simulink model "SMC_network"  (R2021a)
settings: Solver=VariableStepAuto  StartTime=0.0  StopTime=5  RelTol=1e-3
values from neighbouring files (symbols this model uses):
  C = 1e-12    [SMCCodes.m]
  eta_d = 1e27    (= 1e+27)    [SMCCodes.m]
  eta_ds = 1e5    (= 100000)    [SMCCodes.m]
  eta_q = 1e27    (= 1e+27)    [SMCCodes.m]
  eta_qs = 1e5    (= 100000)    [SMCCodes.m]
  g = -10e14    (= -1e+15)    [SMCCodes.m]
  gs = -1/Lt    (= -99.6909580301)    [SMCCodes.m]
  L = 100e-3    (= 0.1)    [SMCCodes.m]
  lambda = 1e10    (= 10000000000)    [SMCCodes.m]
  Lf = 10e-3    (= 0.01)    [SMCCodes.m]
  Lg = 0    [SMCCodes.m]
  Ll = 31e-6    (= 3.1e-05)    [SMCCodes.m]
  phi = 0.01    [SMCCodes.m]
  R = 4.33    [SMCCodes.m]
  Rf = 40e-3    (= 0.04)    [SMCCodes.m]
  RL = 0.1    [SMCCodes.m]
  Ts = 0.50e-5    (= 5e-06)    [SMCCodes.m]
undefined symbols (not defined in the file or in its folder): Ion, Lithium, sigbuilder_block
libraries: spsMeanLib x47, spsSeriesRLCBranchLib x23, simulink x22, spsFirstOrderFilterLib x10, spsIGBTDiodeLib x8, pid_lib x8, spsPWMGeneratorDCDCLib x8, spsabctodq0Lib x7, spsThreePhaseVIMeasurementLib x6, spsCurrentMeasurementLib x4, spsDiodeLib x4, spsIGBTLib x4
(part 1 of 3)
settings Model: SimulationMode=accelerator  Creator=Mori  LastModifiedBy=Mori
settings SolverCC: ZeroCrossAlgorithm=Adaptive
settings OptimizationCC: AccelVerboseBuild=on
settings DebuggingCC: MaskedZcDiagnostic=none  IgnoredZcDiagnostic=none  ModelReferenceExtraNoncontSigs=none

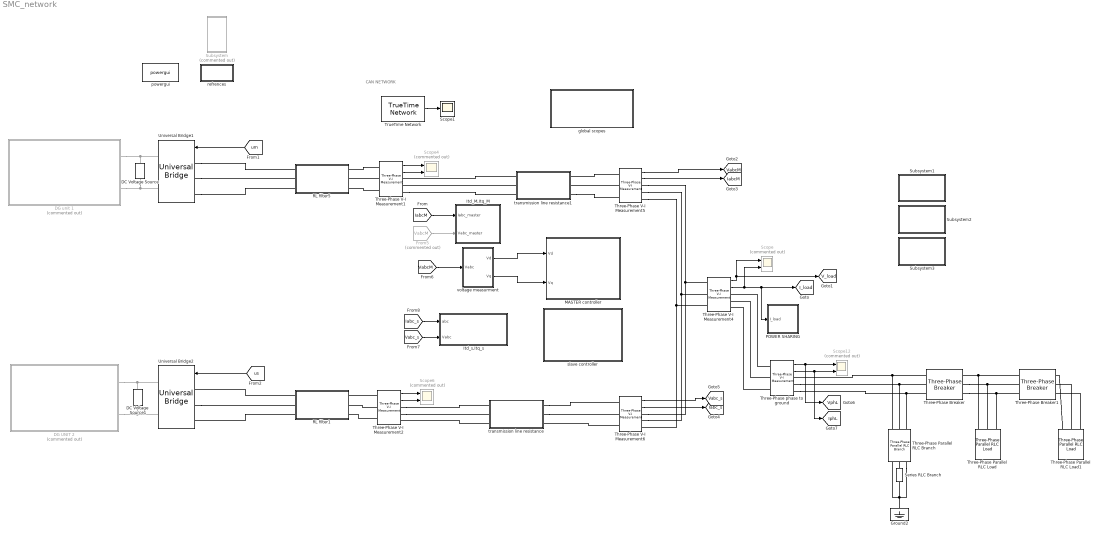
== system SMC_network ==
  note: CAN NETWORK
  DC Voltage Source : spsDCVoltageSourceLib/DC Voltage Source  Amplitude=1000  Measurements=None
  DC Voltage Source1 : spsDCVoltageSourceLib/DC Voltage Source  Amplitude=1000  Measurements=None
  DG UNIT 2 : Subsystem  Commented=on
  DG unit 1 : Subsystem  Commented=on
  From5 : From  Commented=on  GotoTag=VabcM  TagVisibility=global
  Ground2 : spsGroundLib/Ground  LConnTagsString=a
  Itd_M,Itq_M : Subsystem
  Itd_s,Itq_s : Subsystem
  MASTER controller : Subsystem
  POWER SHARING : Subsystem
  RL filter1 : Subsystem
  RL filter5 : Subsystem
  Scope{,4,6,12} (4 alike) : Scope  Commented=on  NumInputPorts=2
  Scope1 : Scope
  Series RLC Branch : spsSeriesRLCBranchLib/Series RLC Branch  LConnTagsString=__new0  RConnTagsString=__new0  BranchType=R  Resistance=0.1  Inductance=1e-3  SetiL0=off  InitialCurrent=0  Capacitance=1e-6  Setx0=off  InitialVoltage=0  Measurements=None
  Subsystem : Subsystem  Commented=on
  Subsystem1 : Subsystem
  Subsystem2 : Subsystem
  Subsystem3 : Subsystem
  Three-Phase Parallel RLC Branch : spsThreePhaseParallelRLCBranchLib/Three-Phase Parallel RLC Branch  LConnTagsString=A|B|C  RConnTagsString=A|B|C  BranchType=RLC  Resistance=R  Inductance=L  Capacitance=C  Measurements=Branch voltages and currents
      settings: SourceProductBaseCode=PS
  Three-Phase Parallel RLC Load : spsThreePhaseParallelRLCLoadLib/Three-Phase Parallel RLC Load  LConnTagsString=A|B|C  Configuration=Y (grounded)  NominalVoltage=380  Vabc=[1e3 1e3 1e3]  Vabcp=[1e3 1e3 1e3]  NominalFrequency=50  UnbalancedPower=off  ActivePower=30e3  InductivePower=5e3  CapacitivePower=0  Pabc=[10e3 9e3 11e3]  QLabc=[100 90 110]  QCabc=[100 90 110]  Pabcp=[10e3 9e3 11e3]  QLabcp=[100 90 110]  QCabcp=[100 90 110]  Measurements=None  LoadType=constant PQ
  Three-Phase Parallel RLC Load1 : spsThreePhaseParallelRLCLoadLib/Three-Phase Parallel RLC Load  LConnTagsString=A|B|C  Configuration=Y (grounded)  NominalVoltage=380  Vabc=[1e3 1e3 1e3]  Vabcp=[1e3 1e3 1e3]  NominalFrequency=50  UnbalancedPower=off  ActivePower=10e3  InductivePower=0  CapacitivePower=0  Pabc=[10e3 9e3 11e3]  QLabc=[100 90 110]  QCabc=[100 90 110]  Pabcp=[10e3 9e3 11e3]  QLabcp=[100 90 110]  QCabcp=[100 90 110]  Measurements=None  LoadType=constant PQ
  Three-Phase V-I Measurement1 : spsThreePhaseVIMeasurementLib/Three-Phase V-I Measurement  VoltageMeasurement=phase-to-phase  SetLabelV=off  LabelV=Vabc  Vpu=off  VpuLL=off  CurrentMeasurement=yes  SetLabelI=off  LabelI=Iabc  Ipu=off  Pbase=100e6  Vbase=500e3  OutputType=Complex  PhasorSimulation=off  PSBequivalent=0
  Three-Phase V-I Measurement2 : spsThreePhaseVIMeasurementLib/Three-Phase V-I Measurement  VoltageMeasurement=phase-to-phase  SetLabelV=off  LabelV=Vabc  Vpu=off  VpuLL=off  CurrentMeasurement=yes  SetLabelI=off  LabelI=Iabc  Ipu=off  Pbase=100e6  Vbase=500e3  OutputType=Complex  PhasorSimulation=off  PSBequivalent=0
  Three-Phase V-I Measurement4 : spsThreePhaseVIMeasurementLib/Three-Phase V-I Measurement  VoltageMeasurement=phase-to-phase  SetLabelV=off  LabelV=Vabc  Vpu=off  VpuLL=off  CurrentMeasurement=yes  SetLabelI=off  LabelI=Iabc  Ipu=off  Pbase=100e6  Vbase=380  OutputType=Complex  PhasorSimulation=off  PSBequivalent=0
  Three-Phase V-I Measurement5 : spsThreePhaseVIMeasurementLib/Three-Phase V-I Measurement  VoltageMeasurement=phase-to-ground  SetLabelV=off  LabelV=Vabc  Vpu=off  VpuLL=off  CurrentMeasurement=yes  SetLabelI=off  LabelI=Iabc  Ipu=off  Pbase=100e6  Vbase=500e3  OutputType=Complex  PhasorSimulation=off  PSBequivalent=0
  Three-Phase V-I Measurement6 : spsThreePhaseVIMeasurementLib/Three-Phase V-I Measurement  VoltageMeasurement=phase-to-ground  SetLabelV=off  LabelV=Vabc  Vpu=off  VpuLL=off  CurrentMeasurement=yes  SetLabelI=off  LabelI=Iabc  Ipu=off  Pbase=100e6  Vbase=500e3  OutputType=Complex  PhasorSimulation=off  PSBequivalent=0
  Three-Phase phase to ground : spsThreePhaseVIMeasurementLib/Three-Phase V-I Measurement  VoltageMeasurement=phase-to-ground  SetLabelV=off  LabelV=Vabc  Vpu=off  VpuLL=off  CurrentMeasurement=yes  SetLabelI=off  LabelI=Iabc  Ipu=off  Pbase=100e6  Vbase=500e3  OutputType=Complex  PhasorSimulation=off  PSBequivalent=0
  Three-Phase Breaker : spsThreePhaseBreakerLib/Three-Phase Breaker  InitialState=open  SwitchA=on  SwitchB=on  SwitchC=on  SwitchTimes=[1,4]  External=off  BreakerResistance=0.001  SnubberResistance=1e6  SnubberCapacitance=inf  Measurements=None
  Three-Phase Breaker1 : spsThreePhaseBreakerLib/Three-Phase Breaker  InitialState=open  SwitchA=on  SwitchB=on  SwitchC=on  SwitchTimes=[2,3]  External=off  BreakerResistance=0.001  SnubberResistance=1e6  SnubberCapacitance=inf  Measurements=None
  TrueTime Network : truetime/TrueTime Network  nwtype=CSMA/AMP (CAN)  nwnbr=1  nnodes=2  rate=10000000  minsize=512  lossprob=0  seed=0  bandwidths=[0.5 0.5]  slotsize=512  schedule=[1 1 2]  memsize=80000  buftype=Common buffer  overflow=Retransmit  dynSchedule=0  miniSlotSize=0  NIT=0  QSortMode=FIFO  sync=0  irtSchedule=0  nrtLength=0  nodeGraph=0  scheduleoutput=on
  Universal Bridge1 : spsUniversalBridgeLib/Universal Bridge  Arms=3  SnubberResistance=1e3  SnubberCapacitance=inf  Device=MOSFET / Diodes  Ron=1e-3  Lon=0  ForwardVoltages="[  0  0  ]"  ForwardVoltage=0  GTOparameters=[ 10e-6 , 20e-6 ]  IGBTparameters=[ 1e-6 , 2e-6 ]  Measurements=None  Measurements_2=None  converterType=Rectifier
  Universal Bridge2 : spsUniversalBridgeLib/Universal Bridge  Arms=3  SnubberResistance=1e3  SnubberCapacitance=inf  Device=MOSFET / Diodes  Ron=1e-3  Lon=0  ForwardVoltages="[  0  0  ]"  ForwardVoltage=0  GTOparameters=[ 10e-6 , 20e-6 ]  IGBTparameters=[ 1e-6 , 2e-6 ]  Measurements=None  Measurements_2=None  converterType=Rectifier
  global scopes : Subsystem
  powergui : spspowerguiLib/powergui  Priority=1  SimulationMode=Discrete  SampleTime=Ts  frequency=60  Iterations=50  frequencyindice=0  Pbase=100e6  ErrMax=1e-4  UnitsV=kV  UnitsW=MW  buscounter=0  FunctionMessages=off  echomessages=off  EnableUseOfTLC=off  CurrentSourceSwitches=off  DisableSnubberDevices=off  DisableRonSwitches=off  DisableVfSwitches=off  DisplayEquations=off  AutomaticDiscreteSolvers=off  SolverType=Tustin/Backward Euler (TBE)  Interpol=off  ExternalGateDelay=off  methode=off  Ts=100  x0status=blocks  SPID=on  SwTol=0  HookPort=off  NonlinearTolerance=1e-4  nMaxIteration=100  ContinueOnMaxIteration=off  RestoreLinks=warning  ResistiveCurrentMeasurement=off  Frange=[0:2:500]  Ylog=off  Xlog=on  ShowGrid=off  save=off  variable=ZData  structure=0  ZoomFFT=off  StartTime=0.0  cycles=1  DisplayStyle=1  fundamental=60  FreqAxis=off  MaxFrequency=1000  frequencyindicesteady=1  RmsSteady=1  display=off
  refrences : Subsystem
  "slave controller " : Subsystem
  transmission line resistance : Subsystem
  transmission line resistance1 : Subsystem
  voltage measurment : Subsystem
  tag scope: I_load=global, IabcM=global, Iabc_s=global, IphL=global, V_load=global, VabcM=global, Vabc_s=global, VphL=global
  wires:
  Three-Phase V-I Measurement4/2 -> Scope/2, POWER SHARING/1(I_load), [I_load]
  Three-Phase V-I Measurement4/1 -> Scope/1, [V_load]
  Three-Phase phase to ground/1 -> [VphL], Scope12/1
  Three-Phase phase to ground/2 -> [IphL], Scope12/2
  [VabcM] -> voltage measurment/1(Vabc)
  [us] -> Universal Bridge2/1
  [um] -> Universal Bridge1/1
  From5/1 -> Itd_M,Itq_M/2(Vabc_master)
  [IabcM] -> Itd_M,Itq_M/1(Iabc_master)
  [Iabc_s] -> Itd_s,Itq_s/1(abc)
  voltage measurment/2(Vq) -> MASTER controller/2(Vq)
  voltage measurment/1(Vd) -> MASTER controller/1(Vd)
  [Vabc_s] -> Itd_s,Itq_s/2(Vabc)
  Three-Phase V-I Measurement1/2 -> Scope4/2
  Three-Phase V-I Measurement1/1 -> Scope4/1
  Three-Phase V-I Measurement2/1 -> Scope6/1
  Three-Phase V-I Measurement2/2 -> Scope6/2
  Three-Phase V-I Measurement6/1 -> [Vabc_s]
  Three-Phase V-I Measurement6/2 -> [Iabc_s]
  Three-Phase V-I Measurement5/1 -> [VabcM]
  Three-Phase V-I Measurement5/2 -> [IabcM]
  TrueTime Network/1 -> Scope1/1
  connections:
  Three-Phase Parallel RLC Branch/RConn3 -- Ground2/LConn1 -- Three-Phase Parallel RLC Branch/RConn1 -- Series RLC Branch/RConn1
  Three-Phase V-I Measurement1/LConn1 -- RL filter5/RConn1
  Three-Phase V-I Measurement1/LConn3 -- RL filter5/RConn3
  Universal Bridge1/LConn1 -- RL filter5/LConn1
  Universal Bridge1/LConn3 -- RL filter5/LConn3
  transmission line resistance1/LConn2 -- Three-Phase V-I Measurement1/RConn2
  Universal Bridge1/LConn2 -- RL filter5/LConn2
  Three-Phase V-I Measurement2/RConn1 -- transmission line resistance/LConn1
  Three-Phase V-I Measurement1/LConn2 -- RL filter5/RConn2
  transmission line resistance/LConn3 -- Three-Phase V-I Measurement2/RConn3
  RL filter1/LConn3 -- Universal Bridge2/LConn3
  Three-Phase V-I Measurement2/LConn2 -- RL filter1/RConn2
  RL filter1/LConn1 -- Universal Bridge2/LConn1
  Universal Bridge2/LConn2 -- RL filter1/LConn2
  Three-Phase V-I Measurement2/LConn3 -- RL filter1/RConn3
  Three-Phase V-I Measurement2/LConn1 -- RL filter1/RConn1
  Three-Phase phase to ground/RConn3 -- Three-Phase Parallel RLC Branch/LConn3 -- Three-Phase Breaker/LConn3
  Three-Phase phase to ground/RConn2 -- Three-Phase Parallel RLC Branch/LConn2 -- Three-Phase Breaker/LConn2
  Three-Phase Breaker/LConn1 -- Three-Phase Parallel RLC Branch/LConn1 -- Three-Phase phase to ground/RConn1
  Series RLC Branch/LConn1 -- Three-Phase Parallel RLC Branch/RConn2
  Three-Phase V-I Measurement1/RConn3 -- transmission line resistance1/LConn3
  Three-Phase V-I Measurement2/RConn2 -- transmission line resistance/LConn2
  transmission line resistance1/LConn1 -- Three-Phase V-I Measurement1/RConn1
  Three-Phase V-I Measurement4/LConn2 -- Three-Phase V-I Measurement6/RConn2 -- Three-Phase V-I Measurement5/RConn2
  transmission line resistance1/RConn3 -- Three-Phase V-I Measurement5/LConn3
  Three-Phase V-I Measurement4/LConn1 -- Three-Phase V-I Measurement6/RConn1 -- Three-Phase V-I Measurement5/RConn1
  Three-Phase V-I Measurement5/RConn3 -- Three-Phase V-I Measurement4/LConn3 -- Three-Phase V-I Measurement6/RConn3
  Three-Phase V-I Measurement5/LConn2 -- transmission line resistance1/RConn2
  Three-Phase V-I Measurement5/LConn1 -- transmission line resistance1/RConn1
  Three-Phase V-I Measurement6/LConn3 -- transmission line resistance/RConn3
  transmission line resistance/RConn2 -- Three-Phase V-I Measurement6/LConn2
  transmission line resistance/RConn1 -- Three-Phase V-I Measurement6/LConn1
  Three-Phase Parallel RLC Load/LConn1 -- Three-Phase Breaker1/LConn1 -- Three-Phase Breaker/RConn1
  Three-Phase Breaker/RConn2 -- Three-Phase Breaker1/LConn2 -- Three-Phase Parallel RLC Load/LConn2
  Three-Phase Breaker/RConn3 -- Three-Phase Breaker1/LConn3 -- Three-Phase Parallel RLC Load/LConn3
  Three-Phase phase to ground/LConn1 -- Three-Phase V-I Measurement4/RConn1
  Three-Phase phase to ground/LConn2 -- Three-Phase V-I Measurement4/RConn2
  Three-Phase phase to ground/LConn3 -- Three-Phase V-I Measurement4/RConn3
  Three-Phase Parallel RLC Load1/LConn1 -- Three-Phase Breaker1/RConn1
  Three-Phase Parallel RLC Load1/LConn2 -- Three-Phase Breaker1/RConn2
  Three-Phase Parallel RLC Load1/LConn3 -- Three-Phase Breaker1/RConn3
  DG unit 1/RConn1 -- DC Voltage Source/RConn1 -- Universal Bridge1/RConn1
  DG unit 1/RConn2 -- DC Voltage Source/LConn1 -- Universal Bridge1/RConn2
  DG UNIT 2/RConn1 -- DC Voltage Source1/RConn1 -- Universal Bridge2/RConn1
  DG UNIT 2/RConn2 -- DC Voltage Source1/LConn1 -- Universal Bridge2/RConn2

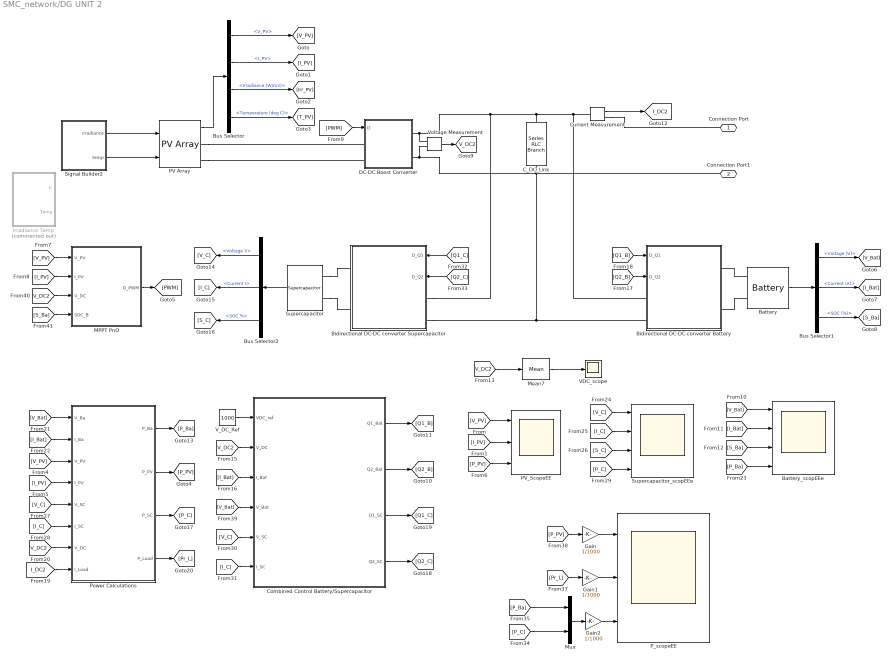
== system SMC_network/DG UNIT 2 ==
  Battery : spsBatteryLib/Battery  BatType=Lithium-Ion  ShowTempParam=off  ThermalPreset=no  ShowAgeParam=off  NomV=750  NomQ=21  SOC=50  Batt_Tr=0.1  PresetModel=on  MaxQ=21  MinV=562.5  FullV=872.9904  Dis_rate=9.1304  R=0.35714  Normal_OP=18.9913  expZone="[810.2894      1.031739]"  current=[9.5 20 28]  Units=Time  Tci=20  NomT=20  T2=-30  MaxQ2=4.8  FullV2=7.1  Normal_OP2=5.655  expZone2="[6.58           1]"  Rca=0.6  ti=2000  Dp=0  Neq0=0  Tsim=1e6  Ta1=25  Qeol=5.4*0.9  Reol=0.013333*1.2  Char_age=[2.3478, 3]  Dis_age=[2.3478, 10]  N1=1500  N2=10500  N3=1000  N4=1400  Ta2=45  N5=950
  "Battery_scopEEe " : Scope  NumInputPorts=4
  Bidirectional DC-DC converter Battery : Subsystem
  Bidirectional DC-DC converter Supercapacitor : Subsystem
  Bus Selector : BusSelector  OutputSignals=V_PV,I_PV,Irradiance (W/m2),Temperature (deg C)
  Bus Selector1 : BusSelector  OutputSignals=Voltage (V),Current (A),SOC (%)
  Bus Selector2 : BusSelector  OutputSignals=Voltage V,Current I,SOC %
  C_DC_Link : spsSeriesRLCBranchLib/Series RLC Branch  LConnTagsString=__new0  RConnTagsString=__new0  BranchType=C  Resistance=1  Inductance=1e-3  SetiL0=off  InitialCurrent=0  Capacitance=500e-6  Setx0=off  InitialVoltage=0  Measurements=None
  Combined Control Battery/Supercapacitor : Subsystem
  Current Measurement : spsCurrentMeasurementLib/Current Measurement  PhasorSimulation=off  OutputType=Complex  PSBequivalent=0
  DC-DC Boost Converter : Subsystem
  Gain : Gain  Gain=1/1000
  Gain1 : Gain  Gain=1/1000
  Gain2 : Gain  Gain=1/1000
  Irradiance Temp : Subsystem  Tag=STV Subsys  Commented=on  LoadFcn=sigbuilder_block('load');  StartFcn=sigbuilder_block('start');  StopFcn=sigbuilder_block('stop');  ClipboardFcn=sigbuilder_block('clipboard');  mask(Sigbuilder block){tuvar=[0:10]}
      mask help: Sigbuilder GUI
      mask init:
      | if ~strcmp(get_param(bdroot(gcbh),'SimulationStatus'),'stopped') tuvar = sigbuilder_block('maskInit'); end
      settings: CopyFcn=sigbuilder_block('copy');  DeleteFcn=sigbuilder_block('delete');  ModelCloseFcn=sigbuilder_block('modelClose');  PreSaveFcn=sigbuilder_block('preSave');  PauseFcn=sigbuilder_block('pause')  ContinueFcn=sigbuilder_block('continue')  NameChangeFcn=sigbuilder_block('namechange');  OpenFcn=sigbuilder_block('open',[216.75 117 531.75 395.25 ]);  CloseFcn=sigbuilder_block('close');
      mask Display: plot(0, 0, 100, 100,[2, 2, 32, 32, 2], [68, 8, 8, 68, 68],[32, 2], [38, 38], [32, 19, 2],[53, 60, 44], [32, 17, 17, 2],[16, 16, 31, 31]);txt = getActiveGroup(gcbh);text(2, 100, txt,'verticalAlignment', 'top');
  MPPT PnO : Subsystem
  Mean7 : spsMeanLib/Mean  Freq=60  Vinit=0  Ts=0
  Mux : Mux  Inputs=2
  PV Array : spsPVArrayLib/PV Array  Npar=3  Nser=30  PlotType=array @ 25 deg.C & specified irradiances  S_vec="[ 1000 800 500  250 ]"  Temp_C_vec="[0 25 50  ]"  ModuleName=Yingli Energy (China) YL250C-30b  PlotWhenSelected=on  Pm=252.815  Ncell=60  Voc=37.6  Isc=9.1  Vm=29.5  Im=8.57  beta_Voc_pc=-0.3  alpha_Isc_pc=0.044  beta_Voc=-0.1128  alpha_Isc=0.004004  IL=9.111  I0=3.084e-11  nI=0.92381  Rsh=475.5958  Rs=0.45532  RobustModel=off  RobustCellTemperature=313.3991  BAL=on  Tc=Tc  Tfilter=5e-5
  PV_ScopeEE : Scope  NumInputPorts=3
  P_scopeEE : Scope  NumInputPorts=3
  Power Calculations : Subsystem
  Signal Builder2 : Subsystem  Tag=STV Subsys  LoadFcn=sigbuilder_block('load');  StartFcn=sigbuilder_block('start');  StopFcn=sigbuilder_block('stop');  ClipboardFcn=sigbuilder_block('clipboard');  mask(Sigbuilder block){tuvar=[0:10]}
      mask help: Simulink:masks:SigbuilderBlock_MD
      mask init:
      | if ~strcmp(get_param(bdroot(gcbh),'SimulationStatus'),'stopped') tuvar = sigbuilder_block('maskInit'); end
      settings: CopyFcn=sigbuilder_block('copy');  DeleteFcn=sigbuilder_block('delete');  ModelCloseFcn=sigbuilder_block('modelClose');  PreSaveFcn=sigbuilder_block('preSave');  PauseFcn=sigbuilder_block('pause');  ContinueFcn=sigbuilder_block('continue');  NameChangeFcn=sigbuilder_block('namechange');  OpenFcn=sigbuilder_block('open',[6 0 1012.5 477.75 ]);  CloseFcn=sigbuilder_block('close');
      mask Display: plot(0, 0, 100, 100,[2, 2, 32, 32, 2], [68, 8, 8, 68, 68],[32, 2], [38, 38], [32, 19, 2],[53, 60, 44], [32, 17, 17, 2],[16, 16, 31, 31]);txt = getActiveGroup(gcbh);text(2, 100, txt,'verticalAlignment', 'top');
  Supercapacitor : spsSupercapacitorLib/Supercapacitor  C=250  Rdc=0.0028  Voltage=820  Ns=1  Np=10  Vinit=820  Temp=25  PresetModel=on  EstParam=off  Nc=1  r=1e-9  epsilon=6.0208e-10  Ich=10  Vstern="[0.161  2.7  7.8]"  Self_dis=on  Ioc=10  Vself="[720  710  701  689]"  demandeplot=off  I=[10 20 100 500]  Units=sec  Vmax=0  If=0  deltaV=0  alpha=0  sec=0
      settings: SourceProductBaseCode=PS
  Supercapacitor_scopEEe : Scope  NumInputPorts=4
  VDC_scope : Scope
  V_DC_Ref : Constant  Value=1000
  Voltage Measurement : spsVoltageMeasurementLib/Voltage Measurement  PhasorSimulation=off  OutputType=Complex  PSBequivalent=0
  Connection Port : PMIOPort  Side=Right
  Connection Port1 : PMIOPort  Port=2  Side=Right
  tag scope: I_DC2=global, V_DC2=global
  wires:
  [P_C] -> Mux/2
  Mux/1 -> Gain2/1
  [P_Ba] -> "Battery_scopEEe "/4
  Mean7/1 -> VDC_scope/1
  [P_Ba] -> Mux/1
  [Pr_L] -> Gain1/1
  [I_Bat] -> Power Calculations/2(I_Ba)
  [P_PV] -> Gain/1
  [I_PV] -> PV_ScopeEE/2
  [V_PV] -> PV_ScopeEE/1
  [I_DC2] -> Power Calculations/8(I_Load)
  [V_Bat] -> Combined Control Battery/Supercapacitor/4(V_Bat)
  Power Calculations/3(P_SC) -> [P_C]
  [V_PV] -> Power Calculations/3(V_PV)
  V_DC_Ref/1 -> Combined Control Battery/Supercapacitor/1(VDC_ref)
  [I_Bat] -> Combined Control Battery/Supercapacitor/3(I_Bat)
  [PWM] -> DC-DC Boost Converter/1(D)
  Bus Selector2/3 -> [S_C]  "<SOC %>"
  [V_DC2] -> Power Calculations/7(V_DC)
  [V_Bat] -> "Battery_scopEEe "/1
  Power Calculations/1(P_Ba) -> [P_Ba]
  [I_C] -> Combined Control Battery/Supercapacitor/6(I_SC)
  [I_Bat] -> "Battery_scopEEe "/2
  Power Calculations/4(P_Load) -> [Pr_L]
  [V_DC2] -> Mean7/1
  [V_PV] -> MPPT PnO/1(V_PV)
  [I_C] -> Power Calculations/6(I_SC)
  [P_PV] -> PV_ScopeEE/3
  [V_Bat] -> Power Calculations/1(V_Ba)
  Current Measurement/1 -> [I_DC2]
  [S_C] -> Supercapacitor_scopEEe/3
  Combined Control Battery/Supercapacitor/3(Q1_SC) -> [Q1_C]
  [S_Ba] -> "Battery_scopEEe "/3
  Bus Selector2/2 -> [I_C]  "<Current I>"
  [P_C] -> Supercapacitor_scopEEe/4
  [V_C] -> Combined Control Battery/Supercapacitor/5("V_SC ")
  Supercapacitor/1 -> Bus Selector2/1
  Bus Selector2/1 -> [V_C]  "<Voltage V>"
  Combined Control Battery/Supercapacitor/2(Q2_Bat) -> [Q2_B]
  [S_Ba] -> MPPT PnO/4(SOC_B)
  [I_C] -> Supercapacitor_scopEEe/2
  [Q2_C] -> Bidirectional DC-DC converter Supercapacitor/2(D_Q2)
  [V_DC2] -> MPPT PnO/3(V_DC)
  [Q1_C] -> Bidirectional DC-DC converter Supercapacitor/1(D_Q1)
  PV Array/1 -> Bus Selector/1
  Bus Selector1/3 -> [S_Ba]  "<SOC (%)>"
  [Q2_B] -> Bidirectional DC-DC converter Battery/2(D_Q2)
  Voltage Measurement/1 -> [V_DC2]
  [Q1_B] -> Bidirectional DC-DC converter Battery/1(D_Q1)
  Battery/1 -> Bus Selector1/1
  [V_DC2] -> Combined Control Battery/Supercapacitor/2(V_DC)
  Bus Selector1/2 -> [I_Bat]  "<Current (A)>"
  Bus Selector1/1 -> [V_Bat]  "<Voltage (V)>"
  [V_C] -> Power Calculations/5(V_SC)
  Bus Selector/4 -> [T_PV]  "<Temperature (deg C)>"
  Combined Control Battery/Supercapacitor/1(Q1_Bat) -> [Q1_B]
  MPPT PnO/1(D_PWM) -> [PWM]
  Bus Selector/3 -> [Irr_PV]  "<Irradiance (W/m2)>"
  Power Calculations/2(P_PV) -> [P_PV]
  [I_PV] -> Power Calculations/4(I_PV)
  Combined Control Battery/Supercapacitor/4(Q2_SC) -> [Q2_C]
  [I_PV] -> MPPT PnO/2(I_PV)
  Bus Selector/2 -> [I_PV]  "<I_PV>"
  Bus Selector/1 -> [V_PV]  "<V_PV>"
  [V_C] -> Supercapacitor_scopEEe/1
  Signal Builder2/1(irradiance) -> PV Array/1
  Signal Builder2/2(temp) -> PV Array/2
  Gain/1 -> P_scopeEE/1
  Gain1/1 -> P_scopeEE/2
  Gain2/1 -> P_scopeEE/3
  connections:
  Bidirectional DC-DC converter Supercapacitor/LConn1 -- Voltage Measurement/LConn1 -- DC-DC Boost Converter/RConn1 -- Bidirectional DC-DC converter Battery/LConn1 -- Current Measurement/LConn1 -- C_DC_Link/LConn1
  Bidirectional DC-DC converter Supercapacitor/LConn2 -- Bidirectional DC-DC converter Battery/LConn2 -- Connection Port1/RConn1 -- C_DC_Link/RConn1 -- Voltage Measurement/LConn2 -- DC-DC Boost Converter/RConn2
  Current Measurement/RConn1 -- Connection Port/RConn1
  Battery/LConn2 -- Bidirectional DC-DC converter Battery/RConn2
  Battery/LConn1 -- Bidirectional DC-DC converter Battery/RConn1
  PV Array/RConn1 -- DC-DC Boost Converter/LConn1
  Supercapacitor/LConn1 -- Bidirectional DC-DC converter Supercapacitor/RConn1
  PV Array/RConn2 -- DC-DC Boost Converter/LConn2
  Supercapacitor/LConn2 -- Bidirectional DC-DC converter Supercapacitor/RConn2

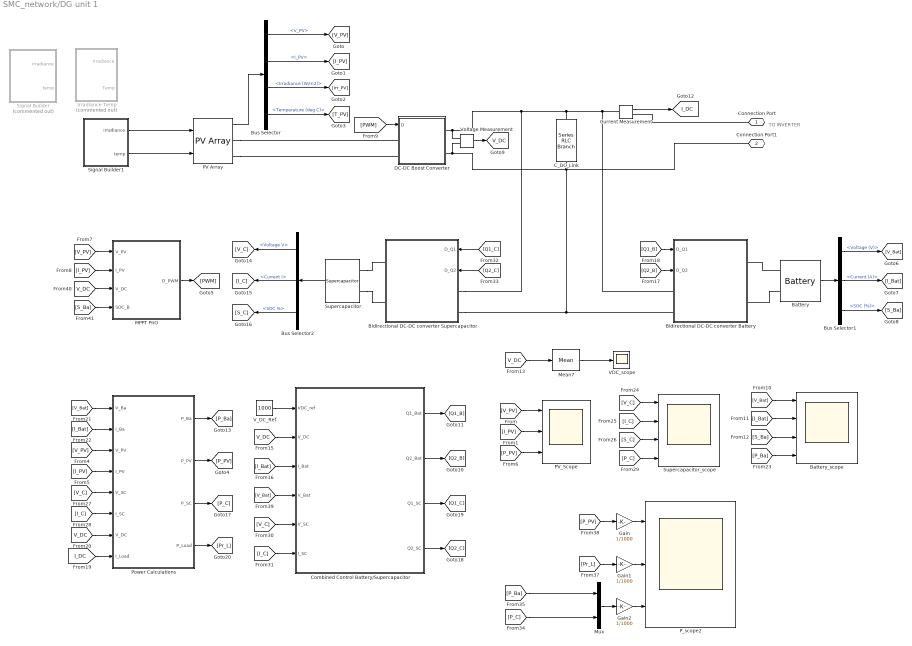
== system SMC_network/DG unit 1 ==
  note: TO INVERTER
  Battery : spsBatteryLib/Battery  BatType=Lithium-Ion  ShowTempParam=off  ThermalPreset=no  ShowAgeParam=off  NomV=750  NomQ=40  SOC=50  Batt_Tr=0.1  PresetModel=on  MaxQ=40  MinV=562.5  FullV=872.9904  Dis_rate=17.3913  R=0.1875  Normal_OP=36.1739  expZone="[810.2894      1.965217]"  current=[17.5 35 52]  Units=Time  Tci=20  NomT=20  T2=-30  MaxQ2=4.8  FullV2=7.1  Normal_OP2=5.655  expZone2="[6.58           1]"  Rca=0.6  ti=2000  Dp=0  Neq0=0  Tsim=1e6  Ta1=25  Qeol=5.4*0.9  Reol=0.013333*1.2  Char_age=[2.3478, 3]  Dis_age=[2.3478, 10]  N1=1500  N2=10500  N3=1000  N4=1400  Ta2=45  N5=950
  "Battery_scope " : Scope  NumInputPorts=4
  Bidirectional DC-DC converter Battery : Subsystem
  Bidirectional DC-DC converter Supercapacitor : Subsystem
  Bus Selector : BusSelector  OutputSignals=V_PV,I_PV,Irradiance (W/m2),Temperature (deg C)
  Bus Selector1 : BusSelector  OutputSignals=Voltage (V),Current (A),SOC (%)
  Bus Selector2 : BusSelector  OutputSignals=Voltage V,Current I,SOC %
  C_DC_Link : spsSeriesRLCBranchLib/Series RLC Branch  LConnTagsString=__new0  RConnTagsString=__new0  BranchType=C  Resistance=1  Inductance=1e-3  SetiL0=off  InitialCurrent=0  Capacitance=500e-6  Setx0=off  InitialVoltage=0  Measurements=None
  Combined Control Battery/Supercapacitor : Subsystem
  Current Measurement : spsCurrentMeasurementLib/Current Measurement  PhasorSimulation=off  OutputType=Complex  PSBequivalent=0
  DC-DC Boost Converter : Subsystem
  Gain : Gain  Gain=1/1000
  Gain1 : Gain  Gain=1/1000
  Gain2 : Gain  Gain=1/1000
  Irradiance Temp : Subsystem  Tag=STV Subsys  Commented=on  LoadFcn=sigbuilder_block('load');  StartFcn=sigbuilder_block('start');  StopFcn=sigbuilder_block('stop');  ClipboardFcn=sigbuilder_block('clipboard');  mask(Sigbuilder block){tuvar=[0:10]}
      mask help: Sigbuilder GUI
      mask init:
      | if ~strcmp(get_param(bdroot(gcbh),'SimulationStatus'),'stopped') tuvar = sigbuilder_block('maskInit'); end
      settings: CopyFcn=sigbuilder_block('copy');  DeleteFcn=sigbuilder_block('delete');  ModelCloseFcn=sigbuilder_block('modelClose');  PreSaveFcn=sigbuilder_block('preSave');  PauseFcn=sigbuilder_block('pause')  ContinueFcn=sigbuilder_block('continue')  NameChangeFcn=sigbuilder_block('namechange');  OpenFcn=sigbuilder_block('open',[0 0 1024.5 518.25 ]);  CloseFcn=sigbuilder_block('close');
      mask Display: plot(0, 0, 100, 100,[2, 2, 32, 32, 2], [68, 8, 8, 68, 68],[32, 2], [38, 38], [32, 19, 2],[53, 60, 44], [32, 17, 17, 2],[16, 16, 31, 31]);txt = getActiveGroup(gcbh);text(2, 100, txt,'verticalAlignment', 'top');
  MPPT PnO : Subsystem
  Mean7 : spsMeanLib/Mean  Freq=60  Vinit=0  Ts=0
  Mux : Mux  Inputs=2
  PV Array : spsPVArrayLib/PV Array  Npar=6  Nser=30  PlotType=array @ 25 deg.C & specified irradiances  S_vec="[ 1000 800 500  250 ]"  Temp_C_vec="[0 25 50  ]"  ModuleName=Yingli Energy (China) YL250P-29b  PlotWhenSelected=on  Pm=250.496  Ncell=60  Voc=38.4  Isc=8.79  Vm=30.4  Im=8.24  beta_Voc_pc=-0.337  alpha_Isc_pc=0.0438  beta_Voc=-0.12941  alpha_Isc=0.00385  IL=8.8005  I0=1.272e-10  nI=0.99849  Rsh=362.5163  Rs=0.42475  RobustModel=off  RobustCellTemperature=313.3991  BAL=on  Tc=Tc  Tfilter=5e-5
  PV_Scope : Scope  NumInputPorts=3
  P_scope2 : Scope  NumInputPorts=3
  Power Calculations : Subsystem
  Signal Builder : Subsystem  Tag=STV Subsys  Commented=on  LoadFcn=sigbuilder_block('load');  StartFcn=sigbuilder_block('start');  StopFcn=sigbuilder_block('stop');  ClipboardFcn=sigbuilder_block('clipboard');  mask(Sigbuilder block){tuvar=[0:10]}
      mask help: Simulink:masks:SigbuilderBlock_MD
      mask init:
      | if ~strcmp(get_param(bdroot(gcbh),'SimulationStatus'),'stopped') tuvar = sigbuilder_block('maskInit'); end
      settings: CopyFcn=sigbuilder_block('copy');  DeleteFcn=sigbuilder_block('delete');  ModelCloseFcn=sigbuilder_block('modelClose');  PreSaveFcn=sigbuilder_block('preSave');  PauseFcn=sigbuilder_block('pause');  ContinueFcn=sigbuilder_block('continue');  NameChangeFcn=sigbuilder_block('namechange');  OpenFcn=sigbuilder_block('open',[6 0 1012.5 477.75 ]);  CloseFcn=sigbuilder_block('close');
      mask Display: plot(0, 0, 100, 100,[2, 2, 32, 32, 2], [68, 8, 8, 68, 68],[32, 2], [38, 38], [32, 19, 2],[53, 60, 44], [32, 17, 17, 2],[16, 16, 31, 31]);txt = getActiveGroup(gcbh);text(2, 100, txt,'verticalAlignment', 'top');
  Signal Builder1 : Subsystem  Tag=STV Subsys  LoadFcn=sigbuilder_block('load');  StartFcn=sigbuilder_block('start');  StopFcn=sigbuilder_block('stop');  ClipboardFcn=sigbuilder_block('clipboard');  mask(Sigbuilder block){tuvar=[0:10]}
      mask help: Simulink:masks:SigbuilderBlock_MD
      mask init:
      | if ~strcmp(get_param(bdroot(gcbh),'SimulationStatus'),'stopped') tuvar = sigbuilder_block('maskInit'); end
      settings: CopyFcn=sigbuilder_block('copy');  DeleteFcn=sigbuilder_block('delete');  ModelCloseFcn=sigbuilder_block('modelClose');  PreSaveFcn=sigbuilder_block('preSave');  PauseFcn=sigbuilder_block('pause');  ContinueFcn=sigbuilder_block('continue');  NameChangeFcn=sigbuilder_block('namechange');  OpenFcn=sigbuilder_block('open',[6 0 1012.5 477.75 ]);  CloseFcn=sigbuilder_block('close');
      mask Display: plot(0, 0, 100, 100,[2, 2, 32, 32, 2], [68, 8, 8, 68, 68],[32, 2], [38, 38], [32, 19, 2],[53, 60, 44], [32, 17, 17, 2],[16, 16, 31, 31]);txt = getActiveGroup(gcbh);text(2, 100, txt,'verticalAlignment', 'top');
  Supercapacitor : spsSupercapacitorLib/Supercapacitor  C=350  Rdc=0.003  Voltage=820  Ns=1  Np=12  Vinit=820  Temp=25  PresetModel=on  EstParam=off  Nc=1  r=1e-9  epsilon=6.0208e-10  Ich=10  Vstern="[0.161  2.7  7.8]"  Self_dis=on  Ioc=10  Vself="[720  710  701  689]"  demandeplot=off  I="[40 50 100  500]"  Units=sec  Vmax=0  If=0  deltaV=0  alpha=0  sec=0
      settings: SourceProductBaseCode=PS
  Supercapacitor_scope : Scope  NumInputPorts=4
  VDC_scope : Scope
  V_DC_Ref : Constant  Value=1000
  Voltage Measurement : spsVoltageMeasurementLib/Voltage Measurement  PhasorSimulation=off  OutputType=Complex  PSBequivalent=0
  Connection Port : PMIOPort  Side=Right
  Connection Port1 : PMIOPort  Port=2  Side=Right
  tag scope: I_DC=global, V_DC=global
  wires:
  [P_C] -> Mux/2
  Bus Selector/2 -> [I_PV]  "<I_PV>"
  [P_PV] -> PV_Scope/3
  Current Measurement/1 -> [I_DC]
  Bus Selector2/1 -> [V_C]  "<Voltage V>"
  [PWM] -> DC-DC Boost Converter/1(D)
  Bus Selector1/2 -> [I_Bat]  "<Current (A)>"
  Bus Selector/4 -> [T_PV]  "<Temperature (deg C)>"
  [I_Bat] -> "Battery_scope "/2
  [V_PV] -> Power Calculations/3(V_PV)
  Power Calculations/4(P_Load) -> [Pr_L]
  [I_PV] -> PV_Scope/2
  Bus Selector1/3 -> [S_Ba]  "<SOC (%)>"
  [Q1_C] -> Bidirectional DC-DC converter Supercapacitor/1(D_Q1)
  Bus Selector2/2 -> [I_C]  "<Current I>"
  Combined Control Battery/Supercapacitor/1(Q1_Bat) -> [Q1_B]
  Combined Control Battery/Supercapacitor/3(Q1_SC) -> [Q1_C]
  [I_PV] -> MPPT PnO/2(I_PV)
  [V_C] -> Combined Control Battery/Supercapacitor/5("V_SC ")
  [Q2_C] -> Bidirectional DC-DC converter Supercapacitor/2(D_Q2)
  [S_C] -> Supercapacitor_scope/3
  [S_Ba] -> "Battery_scope "/3
  Battery/1 -> Bus Selector1/1
  Bus Selector1/1 -> [V_Bat]  "<Voltage (V)>"
  Bus Selector/3 -> [Irr_PV]  "<Irradiance (W/m2)>"
  [Q1_B] -> Bidirectional DC-DC converter Battery/1(D_Q1)
  [I_Bat] -> Power Calculations/2(I_Ba)
  Bus Selector/1 -> [V_PV]  "<V_PV>"
  [V_Bat] -> Power Calculations/1(V_Ba)
  [V_DC] -> Power Calculations/7(V_DC)
  [I_C] -> Combined Control Battery/Supercapacitor/6(I_SC)
  [V_Bat] -> Combined Control Battery/Supercapacitor/4(V_Bat)
  Power Calculations/3(P_SC) -> [P_C]
  [V_DC] -> Mean7/1
  Supercapacitor/1 -> Bus Selector2/1
  Power Calculations/2(P_PV) -> [P_PV]
  Bus Selector2/3 -> [S_C]  "<SOC %>"
  [V_PV] -> MPPT PnO/1(V_PV)
  PV Array/1 -> Bus Selector/1
  [P_Ba] -> Mux/1
  [V_DC] -> MPPT PnO/3(V_DC)
  [V_C] -> Supercapacitor_scope/1
  [I_DC] -> Power Calculations/8(I_Load)
  Combined Control Battery/Supercapacitor/4(Q2_SC) -> [Q2_C]
  [Q2_B] -> Bidirectional DC-DC converter Battery/2(D_Q2)
  Combined Control Battery/Supercapacitor/2(Q2_Bat) -> [Q2_B]
  Mux/1 -> Gain2/1
  MPPT PnO/1(D_PWM) -> [PWM]
  Voltage Measurement/1 -> [V_DC]
  [S_Ba] -> MPPT PnO/4(SOC_B)
  [P_Ba] -> "Battery_scope "/4
  [I_Bat] -> Combined Control Battery/Supercapacitor/3(I_Bat)
  [P_PV] -> Gain/1
  [V_DC] -> Combined Control Battery/Supercapacitor/2(V_DC)
  [P_C] -> Supercapacitor_scope/4
  Mean7/1 -> VDC_scope/1
  [I_PV] -> Power Calculations/4(I_PV)
  [I_C] -> Supercapacitor_scope/2
  [Pr_L] -> Gain1/1
  Power Calculations/1(P_Ba) -> [P_Ba]
  [V_C] -> Power Calculations/5(V_SC)
  [V_Bat] -> "Battery_scope "/1
  [V_PV] -> PV_Scope/1
  [I_C] -> Power Calculations/6(I_SC)
  V_DC_Ref/1 -> Combined Control Battery/Supercapacitor/1(VDC_ref)
  Signal Builder1/2(temp) -> PV Array/2
  Signal Builder1/1(irradiance) -> PV Array/1
  Gain/1 -> P_scope2/1
  Gain1/1 -> P_scope2/2
  Gain2/1 -> P_scope2/3
  connections:
  Bidirectional DC-DC converter Supercapacitor/LConn2 -- Bidirectional DC-DC converter Battery/LConn2 -- Connection Port1/RConn1 -- Voltage Measurement/LConn2 -- DC-DC Boost Converter/RConn2 -- C_DC_Link/RConn1
  C_DC_Link/LConn1 -- Current Measurement/LConn1 -- Bidirectional DC-DC converter Battery/LConn1 -- Bidirectional DC-DC converter Supercapacitor/LConn1 -- Voltage Measurement/LConn1 -- DC-DC Boost Converter/RConn1
  Supercapacitor/LConn1 -- Bidirectional DC-DC converter Supercapacitor/RConn1
  PV Array/RConn1 -- DC-DC Boost Converter/LConn1
  Connection Port/RConn1 -- Current Measurement/RConn1
  PV Array/RConn2 -- DC-DC Boost Converter/LConn2
  Supercapacitor/LConn2 -- Bidirectional DC-DC converter Supercapacitor/RConn2
  Battery/LConn2 -- Bidirectional DC-DC converter Battery/RConn2
  Battery/LConn1 -- Bidirectional DC-DC converter Battery/RConn1

== system SMC_network/Itd_M,Itq_M ==
  Iabc_master : Inport
  Vabc_master : Inport  Port=2
  Demux1 : Demux  Outputs=3
  Demux2 : Demux  Commented=on  Outputs=3
  Goto : Goto  Commented=on  GotoTag=Vd_m  TagVisibility=global
  Goto1 : Goto  Commented=on  GotoTag=Vq_m  TagVisibility=global
  Scope1 : Scope  Commented=on  NumInputPorts=2
  Scope4 : Scope  Commented=on  NumInputPorts=2
  Terminator1 : Terminator
  Terminator2 : Terminator  Commented=on
  abc to dq0 : spsabctodq0Lib/abc to dq0  Alignment=90 degrees behind phase A axis
  abc to dq1 : spsabctodq0Lib/abc to dq0  Commented=on  Alignment=90 degrees behind phase A axis
  tag scope: Itd_M=global, Itq_M=global
  wires:
  Demux1/2 -> Scope4/2, [Itq_M]
  [phase] -> abc to dq1/2, abc to dq0/2
  Demux1/1 -> [Itd_M], Scope4/1
  Demux1/3 -> Terminator1/1
  Iabc_master/1 -> abc to dq0/1
  Demux2/1 -> Scope1/1, Goto/1
  Demux2/2 -> Scope1/2, Goto1/1
  Demux2/3 -> Terminator2/1
  Vabc_master/1 -> abc to dq1/1
  abc to dq0/1 -> Demux1/1
  abc to dq1/1 -> Demux2/1

== system SMC_network/Itd_s,Itq_s ==
  abc : Inport
  Vabc : Inport  Port=2
  Demux : Demux  Outputs=3
  Demux1 : Demux  Outputs=3
  Terminator : Terminator
  Terminator1 : Terminator
  abc to dq0 : spsabctodq0Lib/abc to dq0  Alignment=90 degrees behind phase A axis
  abc to dq1 : spsabctodq0Lib/abc to dq0  Alignment=90 degrees behind phase A axis
  tag scope: Itd_s=global, Itq_s=global, Vds=global, Vqs=global
  wires:
  abc/1 -> abc to dq0/1
  Demux1/3 -> Terminator1/1
  Demux1/1 -> [Itd_s]
  [phase] -> abc to dq0/2
  Demux1/2 -> [Itq_s]
  abc to dq0/1 -> Demux1/1
  Demux/1 -> [Vds]
  Demux/2 -> [Vqs]
  Vabc/1 -> abc to dq1/1
  Demux/3 -> Terminator/1
  [phase] -> abc to dq1/2
  abc to dq1/1 -> Demux/1

== system SMC_network/MASTER controller ==
  Vd : Inport
  Vq : Inport  Port=2
  2OSMC first layer : Subsystem
  Demux : Demux  Outputs=3
  SVPWM Generator (2-Level : spsSVPWMGenerator2LevelLib/SVPWM Generator (2-Level)  InputType=alpha-beta components  SwitchingPattern=Pattern #1  Fc=10000  ParUref=[0.4 0 50]  Ts=0
      settings: SourceProductBaseCode=PS
  Scope : Scope  Commented=on
  Scope1 : Scope  Commented=on  NumInputPorts=2
  Scope2 : Scope  Commented=on  NumInputPorts=2
  Terminator : Terminator
  dq0 to Alpha-Beta Zero : spsdq0toAlphaBetaZeroLib/dq0 to Alpha-Beta-Zero  Alignment=90 degrees behind phase A axis
      settings: SourceProductBaseCode=PS
  tag scope: um=global
  wires:
  Demux/3 -> Terminator/1
  [phase] -> dq0 to Alpha-Beta Zero/2
  2OSMC first layer/1(Udq) -> Scope1/2, dq0 to Alpha-Beta Zero/1
  dq0 to Alpha-Beta Zero/1 -> Scope1/1, Demux/1
  SVPWM Generator (2-Level/1 -> [um], Scope/1
  Demux/1 -> SVPWM Generator (2-Level/1
  Demux/2 -> SVPWM Generator (2-Level/2
  Vd/1 -> Scope2/1, 2OSMC first layer/1(Vd)
  Vq/1 -> 2OSMC first layer/2(Vq), Scope2/2

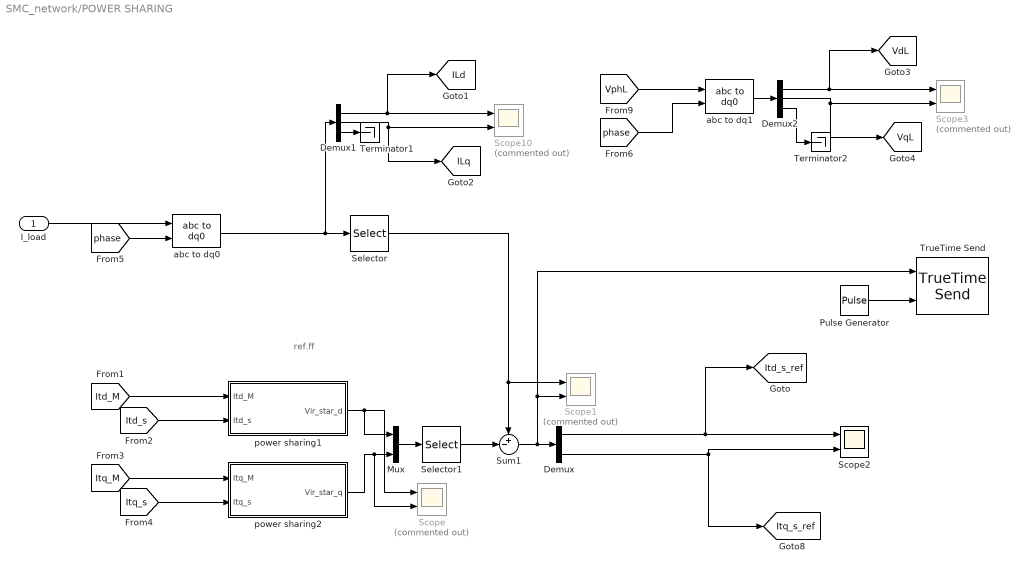
== system SMC_network/POWER SHARING ==
  note: ref.ff
  I_load : Inport
  Demux : Demux  Outputs=2
  Demux1 : Demux  Outputs=3
  Demux2 : Demux  Outputs=3
  Mux : Mux  Inputs=2
  Pulse Generator : DiscretePulseGenerator  PulseType=Time based  Period=1/1000  PulseWidth=25
  Scope{,1,3,10} (4 alike) : Scope  Commented=on  NumInputPorts=2
  Scope2 : Scope  NumInputPorts=2
  Selector : Selector  InputPortWidth=3  IndexOptions=Index vector (dialog)  Indices=[1 2]  OutputSizes=1
  Selector1 : Selector  InputPortWidth=2  IndexOptions=Index vector (dialog)  Indices=[1 2]  OutputSizes=1
  Sum1 : Sum  Inputs=+-|
  Terminator1 : Terminator
  Terminator2 : Terminator
  TrueTime Send : truetime/TrueTime Send  trigger=rising  nwnbr=1  sender=1  indim=2  recsource=internal  receiver=1  lengthsource=internal  length=512  priosource=internal  prio=1  msgIDsource=internal  msgID=0  dynamicSegment=dynamic
  abc to dq0 : spsabctodq0Lib/abc to dq0  Alignment=90 degrees behind phase A axis
  abc to dq1 : spsabctodq0Lib/abc to dq0  Alignment=90 degrees behind phase A axis
  power sharing1 : MATLAB Function  TreatAsAtomicUnit=on
  power sharing2 : MATLAB Function  TreatAsAtomicUnit=on
  tag scope: ILd=global, ILq=global, Itd_s_ref=global, Itq_s_ref=global, VdL=global, VqL=global
  wires:
  I_load/1 -> abc to dq0/1
  [phase] -> abc to dq0/2
  power sharing1/1(Vir_star_d) -> Mux/1, Scope/1
  power sharing2/1(Vir_star_q) -> Scope/2, Mux/2
  Sum1/1 -> TrueTime Send/1, Scope1/2, Demux/1
  Mux/1 -> Selector1/1
  Selector1/1 -> Sum1/2
  Demux1/1 -> [ILd], Scope10/1
  Demux1/2 -> Scope10/2, [ILq]
  Demux1/3 -> Terminator1/1
  [Itd_M] -> power sharing1/1(Itd_M)
  [Itd_s] -> power sharing1/2(Itd_s)
  [Itq_M] -> power sharing2/1(Itq_M)
  [Itq_s] -> power sharing2/2(Itq_s)
  Selector/1 -> Scope1/1, Sum1/1
  abc to dq0/1 -> Selector/1, Demux1/1
  [VphL] -> abc to dq1/1
  [phase] -> abc to dq1/2
  abc to dq1/1 -> Demux2/1
  Demux2/3 -> Terminator2/1
  Demux2/2 -> Scope3/2, [VqL]
  Demux2/1 -> Scope3/1, [VdL]
  Demux/1 -> [Itd_s_ref], Scope2/1
  Demux/2 -> [Itq_s_ref], Scope2/2
  Pulse Generator/1 -> TrueTime Send/2

== system SMC_network/RL filter1 ==
  Three-Phase Series RLC Branch : spsThreePhaseSeriesRLCBranchLib/Three-Phase Series RLC Branch  LConnTagsString=A|B|C  RConnTagsString=A|B|C  BranchType=RL  Resistance=Rf  Inductance=Lf  Capacitance=1e-6  Measurements=None
  Load7 : PMIOPort  Side=Right
  Load8 : PMIOPort  Port=2  Side=Left
  Load9 : PMIOPort  Port=3  Side=Left
  Load10 : PMIOPort  Port=4  Side=Right
  Load11 : PMIOPort  Port=5  Side=Left
  Load12 : PMIOPort  Port=6  Side=Right
  connections:
  Load8/RConn1 -- Three-Phase Series RLC Branch/LConn1
  Load11/RConn1 -- Three-Phase Series RLC Branch/LConn3
  Load9/RConn1 -- Three-Phase Series RLC Branch/LConn2
  Load10/RConn1 -- Three-Phase Series RLC Branch/RConn2
  Load7/RConn1 -- Three-Phase Series RLC Branch/RConn1
  Load12/RConn1 -- Three-Phase Series RLC Branch/RConn3

== system SMC_network/RL filter5 ==
  Three-Phase Series RLC Branch : spsThreePhaseSeriesRLCBranchLib/Three-Phase Series RLC Branch  LConnTagsString=A|B|C  RConnTagsString=A|B|C  BranchType=RL  Resistance=Rf  Inductance=Lf  Capacitance=1e-6  Measurements=None
  Load7 : PMIOPort  Side=Right
  Load8 : PMIOPort  Port=2  Side=Left
  Load9 : PMIOPort  Port=3  Side=Left
  Load10 : PMIOPort  Port=4  Side=Right
  Load11 : PMIOPort  Port=5  Side=Left
  Load12 : PMIOPort  Port=6  Side=Right
  connections:
  Load12/RConn1 -- Three-Phase Series RLC Branch/RConn3
  Load7/RConn1 -- Three-Phase Series RLC Branch/RConn1
  Load10/RConn1 -- Three-Phase Series RLC Branch/RConn2
  Load9/RConn1 -- Three-Phase Series RLC Branch/LConn2
  Load11/RConn1 -- Three-Phase Series RLC Branch/LConn3
  Load8/RConn1 -- Three-Phase Series RLC Branch/LConn1

== system SMC_network/Subsystem ==
  Bus Selector : BusSelector  Commented=on  OutputSignals=V_PV,I_PV
  Bus Selector1 : BusSelector  Commented=on  OutputSignals=V_PV,I_PV
  PV Array : spsPVArrayLib/PV Array  Commented=on  Npar=6  Nser=28  PlotType=array @ 25 deg.C & specified irradiances  S_vec="[ 1000   250 ]"  Temp_C_vec="[0 25 50  ]"  ModuleName=Yingli Energy (China) YL250C-30b  PlotWhenSelected=on  Pm=252.815  Ncell=60  Voc=37.6  Isc=9.1  Vm=29.5  Im=8.57  beta_Voc_pc=-0.3  alpha_Isc_pc=0.044  beta_Voc=-0.1128  alpha_Isc=0.004004  IL=9.111  I0=3.084e-11  nI=0.92381  Rsh=475.5958  Rs=0.45532  RobustModel=off  RobustCellTemperature=313.3991  BAL=on  Tc=Tc  Tfilter=5e-5
  PV Array1 : spsPVArrayLib/PV Array  Commented=on  Npar=3  Nser=28  PlotType=array @ 25 deg.C & specified irradiances  S_vec=[ 1000 800 500 250 ]  Temp_C_vec="[0 25 50  ]"  ModuleName=Yingli Energy (China) YL250C-30b  PlotWhenSelected=on  Pm=252.815  Ncell=60  Voc=37.6  Isc=9.1  Vm=29.5  Im=8.57  beta_Voc_pc=-0.3  alpha_Isc_pc=0.044  beta_Voc=-0.1128  alpha_Isc=0.004004  IL=9.111  I0=3.084e-11  nI=0.92381  Rsh=475.5958  Rs=0.45532  RobustModel=off  RobustCellTemperature=313.3991  BAL=on  Tc=Tc  Tfilter=5e-5
  Radiation : Constant  Commented=on  Value=1000
  Radiation1 : Constant  Commented=on  Value=1000
  Temperature : Constant  Commented=on  Value=25
  Temperature1 : Constant  Commented=on  Value=25
  Vpv1 : Scope  Commented=on  NumInputPorts=2
  Vpv2 : Scope  Commented=on  NumInputPorts=2
  boost converter : Subsystem  Commented=on
      settings: PortSchema="{\"entries\":[{\"content\":{\"sides\":[{\"content\":{\"connectorIds\":[\"LConn1\",\"LConn2\"]},\"type\":\"ConnectorPlacement.EquallySpacedRectSide\",\"uuid\":\"17560fca-b081-4b2c-8564-d6b75f1e78ac\"},{\"content\":{\"connectorIds\":[\"RConn1\",\"RConn2\"],\"side\":\"RIGHT\"},\"type\":\"ConnectorPlacement.EquallySpacedRectSide\",\"uuid\":\"eac739bb-0900-4bda-9654-1f3f93e38410\"},{\"content\":{\"connectorIds\":[\"In1\",\"In2\"],\"side\":\"TOP\"},\"type\":\"ConnectorPlacement.EquallySpacedRectSide\",\"uuid\":\"f9fcd845-384d-4c9c-96fa-60701e43d6a4\"}]},\"type\":\"ConnectorPlacement.EquallySpacedConnector\",\"uuid\":\"6c9b23ff-5189-4090-aced-6ff0c030958c\"}],\"packageUris\":[\"http://schema.mathworks.com/mf0/Connector/R2020b\"],\"version\":\"1.0\"}"
  boost converter1 : Subsystem  Commented=on
      settings: PortSchema="{\"entries\":[{\"content\":{\"sides\":[{\"content\":{\"connectorIds\":[\"LConn1\",\"LConn2\"]},\"type\":\"ConnectorPlacement.EquallySpacedRectSide\",\"uuid\":\"17560fca-b081-4b2c-8564-d6b75f1e78ac\"},{\"content\":{\"connectorIds\":[\"RConn1\",\"RConn2\"],\"side\":\"RIGHT\"},\"type\":\"ConnectorPlacement.EquallySpacedRectSide\",\"uuid\":\"eac739bb-0900-4bda-9654-1f3f93e38410\"},{\"content\":{\"connectorIds\":[\"In1\",\"In2\"],\"side\":\"TOP\"},\"type\":\"ConnectorPlacement.EquallySpacedRectSide\",\"uuid\":\"f9fcd845-384d-4c9c-96fa-60701e43d6a4\"}]},\"type\":\"ConnectorPlacement.EquallySpacedConnector\",\"uuid\":\"6c9b23ff-5189-4090-aced-6ff0c030958c\"}],\"packageUris\":[\"http://schema.mathworks.com/mf0/Connector/R2020b\"],\"version\":\"1.0\"}"
  + : PMIOPort  Side=Right
  - : PMIOPort  Port=2  Side=Right
  +1 : PMIOPort  Port=3  Side=Right
  -1 : PMIOPort  Port=4  Side=Right
  wires:
  Radiation/1 -> PV Array/1
  Bus Selector1/1 -> Vpv2/1, boost converter1/1(,Vpv)  "<V_PV>"
  PV Array/1 -> Bus Selector/1
  Radiation1/1 -> PV Array1/1
  Temperature/1 -> PV Array/2
  PV Array1/1 -> Bus Selector1/1
  Bus Selector/1 -> Vpv1/1, boost converter/1(,Vpv)  "<V_PV>"
  Temperature1/1 -> PV Array1/2
  Bus Selector/2 -> Vpv1/2, boost converter/2("Ipv ")  "<I_PV>"
  Bus Selector1/2 -> Vpv2/2, boost converter1/2("Ipv ")  "<I_PV>"
  connections:
  PV Array/RConn2 -- boost converter/LConn2
  PV Array1/RConn2 -- boost converter1/LConn2
  boost converter/LConn1 -- PV Array/RConn1
  boost converter1/LConn1 -- PV Array1/RConn1
  boost converter1/RConn1 -- +1/RConn1
  boost converter1/RConn2 -- -1/RConn1
  boost converter/RConn1 -- +/RConn1
  boost converter/RConn2 -- -/RConn1

== system SMC_network/Subsystem1 ==
  MATLAB Function : MATLAB Function  TreatAsAtomicUnit=on
  MATLAB Function1 : MATLAB Function  TreatAsAtomicUnit=on
  tag scope: P_L=global, Q_L=global
  wires:
  [VdL] -> MATLAB Function/2(Vd), MATLAB Function1/2(Vd)
  MATLAB Function1/1(QL) -> [Q_L]
  MATLAB Function/1(pL) -> [P_L]
  [ILq] -> MATLAB Function1/1(ILq)
  [ILd] -> MATLAB Function/1(ILd)

== system SMC_network/Subsystem2 ==
  MATLAB Function : MATLAB Function  TreatAsAtomicUnit=on
  MATLAB Function1 : MATLAB Function  TreatAsAtomicUnit=on
  tag scope: P_M=global, Q_M=global
  wires:
  MATLAB Function/1(p_M) -> [P_M]
  MATLAB Function1/1(Q_M) -> [Q_M]
  [Itq_M] -> MATLAB Function1/1(Itq_M)
  [Vd] -> MATLAB Function1/2(Vd), MATLAB Function/2(Vd)
  [Itd_M] -> MATLAB Function/1(Itd_M)

== system SMC_network/Subsystem3 ==
  MATLAB Function : MATLAB Function  TreatAsAtomicUnit=on
  MATLAB Function1 : MATLAB Function  TreatAsAtomicUnit=on
  tag scope: P_S=global, Q_S=global
  wires:
  [Itd_s] -> MATLAB Function/1(Itd_s)
  [Vds] -> MATLAB Function/2(Vds), MATLAB Function1/2(Vds)
  [Itq_s] -> MATLAB Function1/1(Itq_s)
  MATLAB Function1/1(Q_S) -> [Q_S]
  MATLAB Function/1(p_S) -> [P_S]

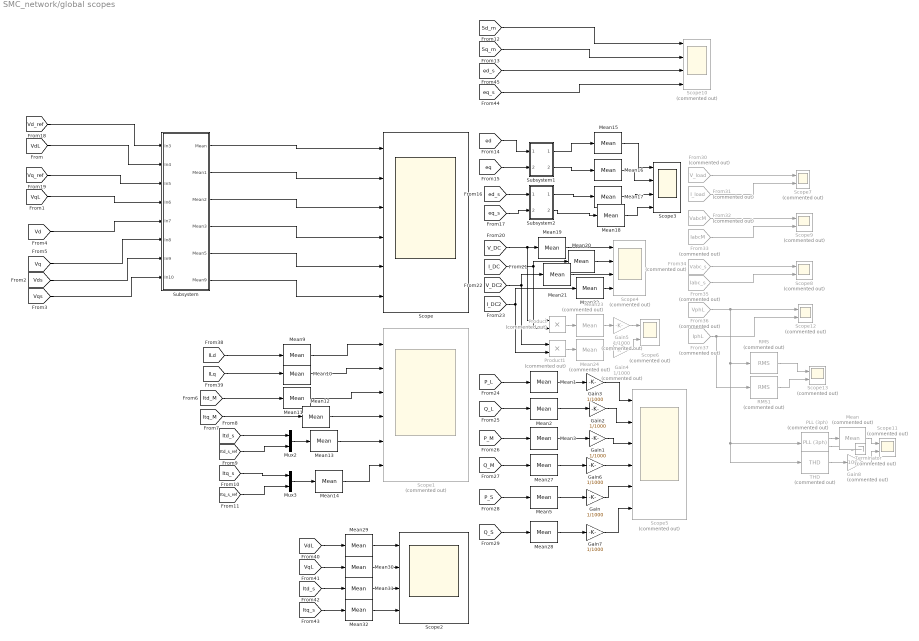
== system SMC_network/global scopes ==
  From30 : From  Commented=on  GotoTag=V_load  TagVisibility=global
  From31 : From  Commented=on  GotoTag=I_load  TagVisibility=global
  From32 : From  Commented=on  GotoTag=VabcM  TagVisibility=global
  From33 : From  Commented=on  GotoTag=IabcM  TagVisibility=global
  From34 : From  Commented=on  GotoTag=Vabc_s  TagVisibility=global
  From35 : From  Commented=on  GotoTag=Iabc_s  TagVisibility=global
  From36 : From  Commented=on  GotoTag=VphL  TagVisibility=global
  From37 : From  Commented=on  GotoTag=IphL  TagVisibility=global
  Gain{,1..3,6..7} (6 alike) : Gain  Gain=1/1000
  Gain4 : Gain  Commented=on  Gain=1/1000
  Gain5 : Gain  Commented=on  Gain=1/1000
  Gain8 : Gain  Commented=on  Gain=100
  Mean : spsMeanLib/Mean  Commented=on  Freq=60  Vinit=0  Ts=0
  Mean{1..3,5,9..22,27..32} (24 alike) : spsMeanLib/Mean  Freq=50  Vinit=0  Ts=0
  Mean23 : spsMeanLib/Mean  Commented=on  Freq=50  Vinit=0  Ts=0
  Mean24 : spsMeanLib/Mean  Commented=on  Freq=50  Vinit=0  Ts=0
  Mux2 : Mux  Inputs=2
  Mux3 : Mux  Inputs=2
  PLL (3ph) : spsPLL3phLib/PLL (3ph)  Commented=on  Fmin=45  Par_Init=[0, 50]  ParK=[180, 3200, 1]  TcD=1e-4  MaxRateChangeFreq=12  FilterCutOffFreq=100  Ts=0  AGC=on
  Product : Product  Commented=on
  Product1 : Product  Commented=on
  RMS : spsRMSLib/RMS  Commented=on  TrueRMS=on  Freq=50  RMSInit=0  Ts=0
  RMS1 : spsRMSLib/RMS  Commented=on  TrueRMS=on  Freq=50  RMSInit=0  Ts=0
  Scope : Scope  NumInputPorts=6
  Scope1 : Scope  Commented=on  NumInputPorts=6
  Scope10 : Scope  Commented=on  NumInputPorts=4
  Scope{6..9,11..13} (7 alike) : Scope  Commented=on  NumInputPorts=2
  Scope2 : Scope  NumInputPorts=4
  Scope3 : Scope  NumInputPorts=4
  Scope4 : Scope  Commented=on  NumInputPorts=4
  Scope5 : Scope  Commented=on  NumInputPorts=6
  Subsystem : Subsystem
  Subsystem1 : Subsystem
  Subsystem2 : Subsystem
  THD : spsTHDLib/THD  Commented=on  Freq=50  Ts=0
      settings: SourceProductBaseCode=PS
  Terminator : Terminator  Commented=on
  wires:
  [Vq_ref] -> Subsystem/3(In5)
  [Itd_s] -> Mux2/1
  [Itd_s_ref] -> Mux2/2
  [Itq_s] -> Mux3/1
  [Itq_s_ref] -> Mux3/2
  [V_DC] -> Product/1, Mean19/1
  [I_DC] -> Product/2, Mean20/1
  [V_DC2] -> Product1/1, Mean21/1
  [I_DC2] -> Mean22/1, Product1/2
  [Q_L] -> Mean2/1
  [P_L] -> Mean1/1
  [P_M] -> Mean3/1
  Product/1 -> Mean23/1
  Product1/1 -> Mean24/1
  From33/1 -> Scope9/2
  From34/1 -> Scope8/1
  From35/1 -> Scope8/2
  From31/1 -> Scope7/2
  From36/1 -> THD/1, PLL (3ph)/1, RMS/1, Scope12/1
  From37/1 -> RMS1/1, Scope12/2
  Mean1/1 -> Gain3/1
  Mean2/1 -> Gain2/1
  Mean5/1 -> Gain/1
  Mean3/1 -> Gain1/1
  Mean19/1 -> Scope4/1
  Mean20/1 -> Scope4/2
  Mean21/1 -> Scope4/3
  Mean22/1 -> Scope4/4
  Mean23/1 -> Gain5/1
  Mean24/1 -> Gain4/1
  From30/1 -> Scope7/1
  From32/1 -> Scope9/1
  [ILd] -> Mean9/1
  [ILq] -> Mean10/1
  [Itd_M] -> Mean11/1
  [Itq_M] -> Mean12/1
  Mux2/1 -> Mean13/1
  Mux3/1 -> Mean14/1
  RMS/1 -> Scope13/1
  RMS1/1 -> Scope13/2
  [VqL] -> Mean30/1
  [VdL] -> Mean29/1
  [Itd_s] -> Mean31/1
  [Itq_s] -> Mean32/1
  Mean29/1 -> Scope2/1
  Mean30/1 -> Scope2/2
  Mean31/1 -> Scope2/3
  Mean32/1 -> Scope2/4
  [ed_s] -> Scope10/3
  [eq_s] -> Scope10/4
  Mean/1 -> Scope11/1
  PLL (3ph)/1 -> Mean/1
  THD/1 -> Gain8/1
  PLL (3ph)/2 -> Terminator/1
  Mean9/1 -> Scope1/1
  Mean10/1 -> Scope1/2
  Mean11/1 -> Scope1/3
  Mean12/1 -> Scope1/4
  Mean13/1 -> Scope1/5
  Mean14/1 -> Scope1/6
  [Sd_m] -> Scope10/1
  [Sq_m] -> Scope10/2
  Mean15/1 -> Scope3/1
  Mean16/1 -> Scope3/2
  Mean17/1 -> Scope3/3
  Mean18/1 -> Scope3/4
  Gain4/1 -> Scope6/2
  Gain5/1 -> Scope6/1
  [Q_M] -> Mean27/1
  Mean27/1 -> Gain6/1
  [P_S] -> Mean5/1
  [Q_S] -> Mean28/1
  Mean28/1 -> Gain7/1
  Gain3/1 -> Scope5/1
  Gain2/1 -> Scope5/2
  Gain6/1 -> Scope5/4
  Gain1/1 -> Scope5/3
  Gain/1 -> Scope5/5
  Gain7/1 -> Scope5/6
  Gain8/1 -> Scope11/2
  [Vd_ref] -> Subsystem/1(In3)
  [VdL] -> Subsystem/2(In4)
  [VqL] -> Subsystem/4(In6)
  [Vd] -> Subsystem/5(In7)
  [Vq] -> Subsystem/6(In8)
  [Vds] -> Subsystem/7(In9)
  [Vqs] -> Subsystem/8(In10)
  Subsystem/1(Mean) -> Scope/1
  Subsystem/2(Mean1) -> Scope/2
  Subsystem/3(Mean2) -> Scope/3
  Subsystem/4(Mean3) -> Scope/4
  Subsystem/5(Mean5) -> Scope/5
  Subsystem/6(Mean9) -> Scope/6
  Subsystem1/1(Out1) -> Mean15/1
  Subsystem1/2(Out2) -> Mean16/1
  Subsystem2/1(Out1) -> Mean17/1
  Subsystem2/2(Out2) -> Mean18/1
  [ed] -> Subsystem1/1(In2)
  [ed_s] -> Subsystem2/1(In1)
  [eq_s] -> Subsystem2/2(In2)
  [eq] -> Subsystem1/2(In1)

== system SMC_network/refrences ==
  Constant1 : Constant  Value=311.1  LockScale=on
  Constant2 : Constant  Value=0  LockScale=on
  Discrete Virtual PLL : Subsystem  DialogController=POWERSYS.PowerSysDialog  mask(Discrete Virtual PLL){Freq=50, Phase=0, Ts=Ts}
      mask prompts: Freq "Frequency (Hz):"; Phase "Phase (degrees):"; Ts "Sample time:"
      mask help:
      | This virtual PLL has no input signal. The block simulates the outputs of an actual PLL by  using the parameters specified in the mask.
      |
      | Output 1: Frequency (Hz)
      | Output 2: Vectorized output  [sin(wt)  cos(wt)]
      | Output 3: wt in rad/s (varying from 0 to 2*pi)
      mask init:
      | power_initmask();
      mask Display: disp('')
  Scope3 : Scope
  Terminator1 : Terminator
  Terminator2 : Terminator
  tag scope: Vd_ref=global, Vq_ref=global, phase=global
  wires:
  Constant1/1 -> [Vd_ref]
  Constant2/1 -> [Vq_ref]
  Discrete Virtual PLL/1(Freq) -> Terminator1/1
  Discrete Virtual PLL/2(Sin_Cos) -> Terminator2/1
  Discrete Virtual PLL/3(wt) -> [phase], Scope3/1
